simulink model "plantFC1"  (Simulink 7.6)
settings: Solver=ode45  StartTime=0.0  StopTime=1000  RelTol=1e-3
libraries: fuzblock x1
settings Model: Creator=kif  LastModifiedBy=kif

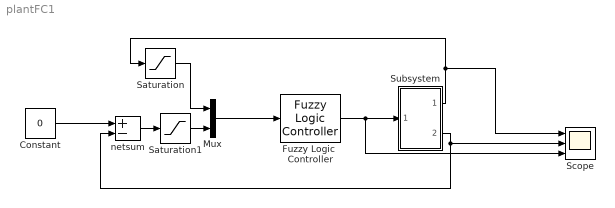
== system plantFC1 ==
  Constant : Constant  Value=0
  Fuzzy Logic  Controller : fuzblock/Fuzzy Logic  Controller  SystemSampleTime=-1  fis=TwoTankFC1
  Mux : Mux  Inputs=2
  Saturation : Saturate  UpperLimit=70  LowerLimit=0
  Saturation1 : Saturate  UpperLimit=70  LowerLimit=-70
  Scope : Scope  NumInputPorts=3
      settings: YMin=-5~-5~0  YMax=5~5~0.5
  Subsystem : Subsystem
  netsum : Sum  Inputs=+-  SaturateOnIntegerOverflow=on  InputSameDT=on  OutDataTypeStr=Inherit: Same as first input
  wires:
  netsum/1 -> Saturation1/1
  Mux/1 -> Fuzzy Logic  Controller/1
  Fuzzy Logic  Controller/1 -> Subsystem/1(In1), Scope/3
  Saturation/1 -> Mux/1
  Saturation1/1 -> Mux/2
  Subsystem/1(Out1) -> Saturation/1, Scope/1
  Subsystem/2(Out2) -> netsum/2, Scope/2
  Constant/1 -> netsum/1

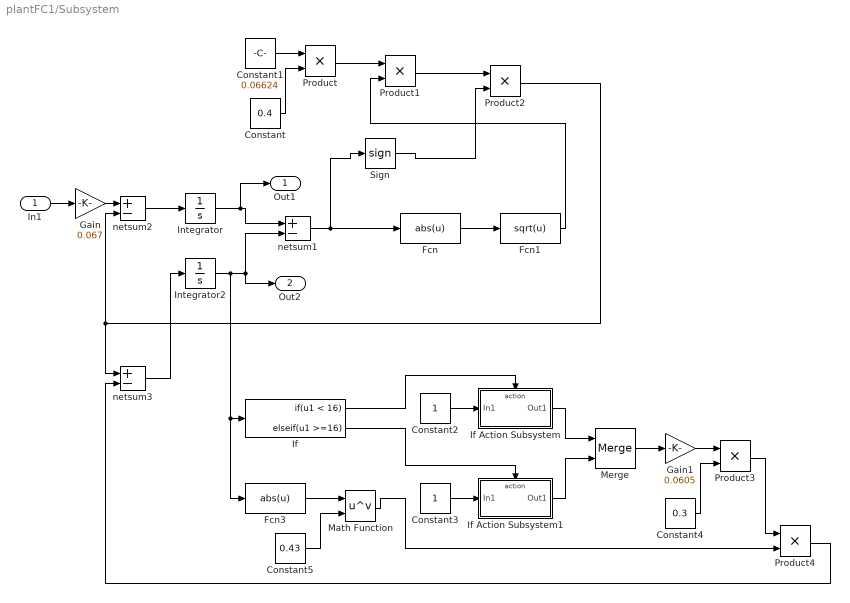
== system plantFC1/Subsystem ==
  In1 : Inport
  Constant : Constant  Value=0.4
  Constant1 : Constant  Value=0.06624
  Constant2 : Constant
  Constant3 : Constant
  Constant4 : Constant  Value=0.3
  Constant5 : Constant  Value=0.43
  Fcn : Fcn  Expr=abs(u)
  Fcn1 : Fcn  Expr=sqrt(u)
  Fcn3 : Fcn  Expr=abs(u)
  Gain : Gain  Gain=0.067
  Gain1 : Gain  Gain=0.0605
  If : If  IfExpression=u1 < 16  ElseIfExpressions=u1 >=16  ShowElse=off
  If Action Subsystem : Subsystem  TreatAsAtomicUnit=on
  If Action Subsystem1 : Subsystem  TreatAsAtomicUnit=on
  Integrator : Integrator  Tag=x1  InitialCondition=0.0001
      settings: AttributesFormatString=%<Tag>
  Integrator2 : Integrator  Tag=x2
      settings: AttributesFormatString=%<Tag>
  Math Function : Math  Operator=pow  SaturateOnIntegerOverflow=on
  Merge : Merge
  Product{,1,3..4} (4 alike) : Product  RndMeth=Zero
  Product2 : Product  Tag=f  RndMeth=Zero
      settings: AttributesFormatString=%<Tag>
  Sign : Signum
  netsum1 : Sum  Inputs=+-  SaturateOnIntegerOverflow=on  InputSameDT=on  OutDataTypeStr=Inherit: Same as first input
  netsum2 : Sum  Inputs=+-  SaturateOnIntegerOverflow=on  InputSameDT=on  OutDataTypeStr=Inherit: Same as first input
  netsum3 : Sum  Inputs=+-  SaturateOnIntegerOverflow=on  InputSameDT=on  OutDataTypeStr=Inherit: Same as first input
  Out1 : Outport
  Out2 : Outport  Port=2
  wires:
  Constant/1 -> Product/2
  Product/1 -> Product1/1
  Integrator/1 -> netsum1/1, Out1/1
  Integrator2/1 -> If/1, Fcn3/1, netsum1/2, Out2/1
  Fcn/1 -> Fcn1/1
  Fcn1/1 -> Product1/2
  netsum1/1 -> Fcn/1, Sign/1
  Constant1/1 -> Product/1
  Product1/1 -> Product2/1
  Sign/1 -> Product2/2
  Gain/1 -> netsum2/1
  Product2/1 -> netsum2/2, netsum3/1
  netsum2/1 -> Integrator/1
  Constant2/1 -> If Action Subsystem/1(In1)
  Constant3/1 -> If Action Subsystem1/1(In1)
  If/2 -> If Action Subsystem1/Action
  If/1 -> If Action Subsystem/Action
  If Action Subsystem/1(Out1) -> Merge/1
  If Action Subsystem1/1(Out1) -> Merge/2
  Merge/1 -> Gain1/1
  Gain1/1 -> Product3/1
  Constant4/1 -> Product3/2
  Fcn3/1 -> Math Function/1
  Product3/1 -> Product4/1
  Math Function/1 -> Product4/2
  Product4/1 -> netsum3/2
  netsum3/1 -> Integrator2/1
  In1/1 -> Gain/1
  Constant5/1 -> Math Function/2

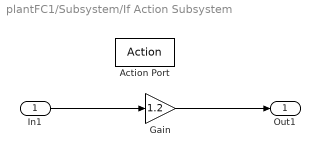
== system plantFC1/Subsystem/If Action Subsystem ==
  In1 : Inport
  Action Port : ActionPort  ActionType=then
  Gain : Gain  Gain=1.2
  Out1 : Outport
  wires:
  In1/1 -> Gain/1
  Gain/1 -> Out1/1

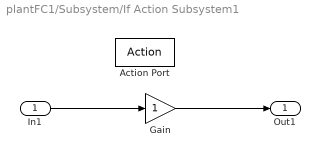
== system plantFC1/Subsystem/If Action Subsystem1 ==
  In1 : Inport
  Action Port : ActionPort  ActionType=elseif
  Gain : Gain
  Out1 : Outport
  wires:
  In1/1 -> Gain/1
  Gain/1 -> Out1/1
